simulink model "lab12_simulink"  (R2024a)
settings: Solver=VariableStepAuto  StartTime=0.0  StopTime=10.0  RelTol=1e-3
settings Model: Creator=Admin  LastModifiedBy=Admin

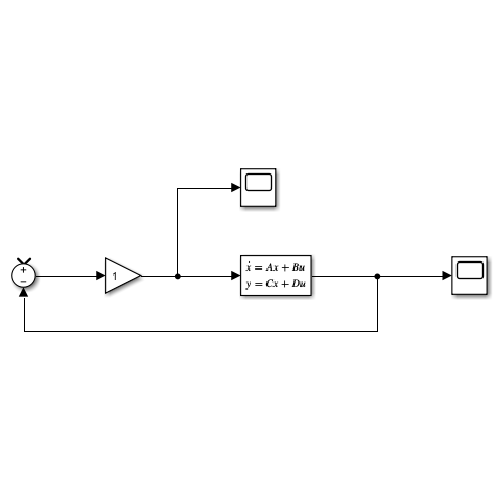
[thumbnail: Simulink's stored preview of the top-level diagram]
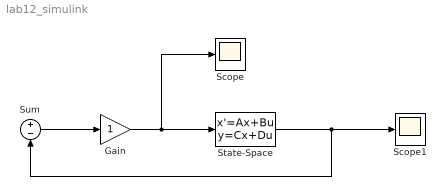
== system lab12_simulink ==
  Gain : Gain
  Scope : Scope
  Scope1 : Scope
  State-Space : StateSpace  InitialCondition=0
  Sum : Sum  Inputs=+-
  wires:
  Gain/1 -> Scope/1, State-Space/1
  State-Space/1 -> Sum/2, Scope1/1
  Sum/1 -> Gain/1
